simulink model "control_loop"  (R2023b)
settings: Solver=ode1  StartTime=0.0  StopTime=30  FixedStep=time_step  RelTol=1e-3
model workspace (MAT data in the model file):
  time_step = 0.002
libraries: simulink x1
settings Model: Creator=danie  LastModifiedBy=danie

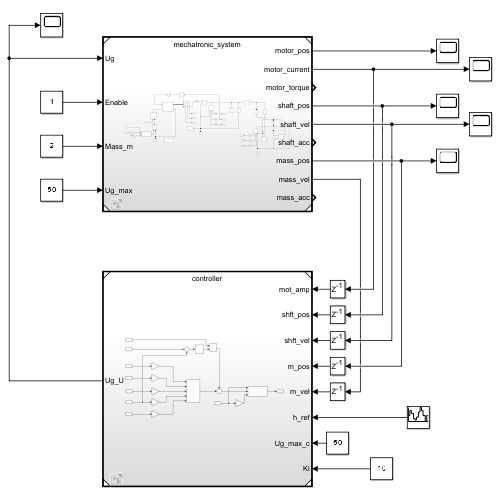
[thumbnail: Simulink's stored preview of the top-level diagram]
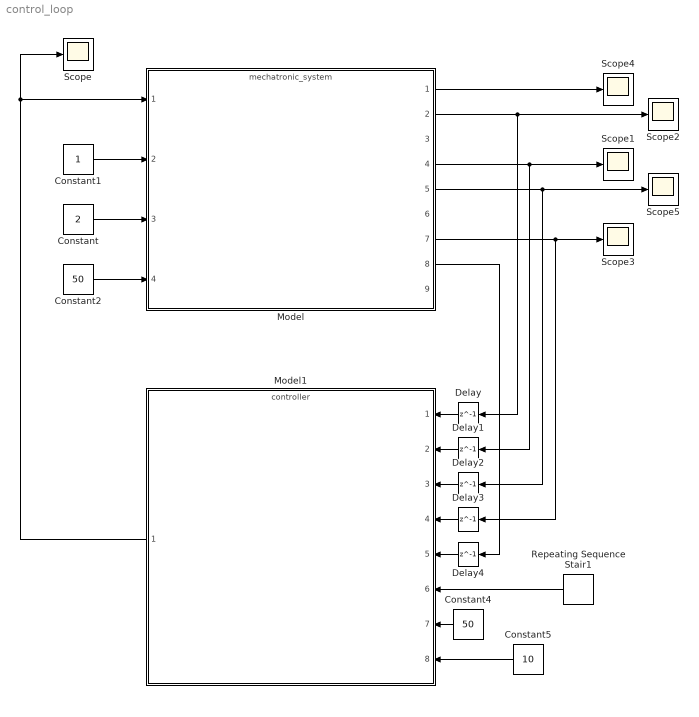
== system control_loop ==
  Constant : Constant  Value=2
  Constant1 : Constant
  Constant2 : Constant  Value=50
  Constant4 : Constant  Value=50
  Constant5 : Constant  Value=10
  Delay{,1..4} (5 alike) : Delay  DelayLength=1  InitialCondition=0
  Model : ModelReference  ModelNameDialog=mechatronic_system.slx  SimulationMode=Normal  ModelReferenceVersion=1.22
  Model1 : ModelReference  ModelNameDialog=controller.slx  SimulationMode=Normal  ModelReferenceVersion=1.27
  Repeating Sequence Stair1 : simulink/Sources/Repeating Sequence Stair  OutValues=[2 4 3 1 0.5 1.5 3.5 5.0 4.0 2.0 0.0 2.0].'  tsamp=25  OutMin=[]  OutMax=[]  OutDataTypeStr=double  OutputDataTypeScalingMode=double  OutDataType=fixdt(0,8)  ConRadixGroup=Best Precision: Vector-wise  OutScaling=2^-12
  Scope{,1..5} (6 alike) : Scope
  wires:
  Model1/1 -> Scope/1, Model/1
  Constant1/1 -> Model/2
  Model/7 -> Delay3/1, Scope3/1
  Model/1 -> Scope4/1
  Model/4 -> Delay1/1, Scope1/1
  Model/2 -> Delay/1, Scope2/1
  Model/5 -> Delay2/1, Scope5/1
  Constant/1 -> Model/3
  Constant2/1 -> Model/4
  Model/8 -> Delay4/1
  Repeating Sequence Stair1/1 -> Model1/6
  Delay/1 -> Model1/1
  Delay1/1 -> Model1/2
  Delay2/1 -> Model1/3
  Delay3/1 -> Model1/4
  Delay4/1 -> Model1/5
  Constant4/1 -> Model1/7
  Constant5/1 -> Model1/8
